simulink model "WP1openloop"  (R2023a)
settings: Solver=ode45  StartTime=0.0  StopTime=100  MaxStep=2  RelTol=1e-14  AbsTol=1e-20
values from neighbouring files (symbols this model uses):
  x1 = x(1)    [WP1.m]    (also in plotSimulationResults.m = x(:, 1))
  x2 = x(2)    [WP1.m]    (also in plotSimulationResults.m = x(:, 2))
settings Model: Creator=giova  LastModifiedBy=giova

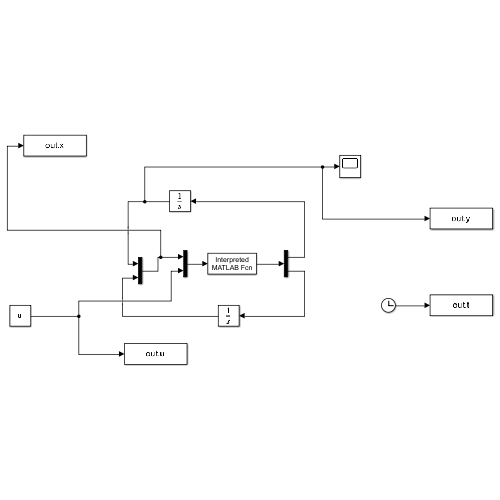
[thumbnail: Simulink's stored preview of the top-level diagram]
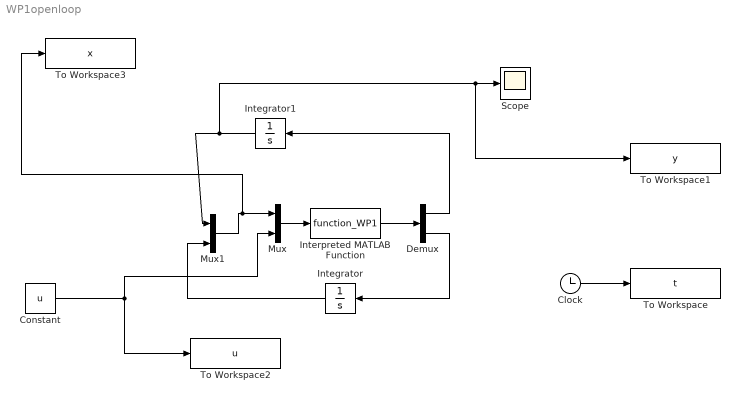
== system WP1openloop ==
  Clock : Clock
  Constant : Constant  Value=u
  Demux : Demux  Outputs=2
  Integrator : Integrator  InitialCondition=x2
  Integrator1 : Integrator  InitialCondition=x1
  Interpreted MATLAB Function : MATLABFcn  MATLABFcn=function_WP1  OutputDimensions=2
  Mux : Mux  Inputs=2
  Mux1 : Mux  Inputs=2
  Scope : Scope
  To Workspace : ToWorkspace  VariableName=t  SampleTime=-1
  To Workspace1 : ToWorkspace  VariableName=y  SampleTime=-1
  To Workspace2 : ToWorkspace  VariableName=u  SampleTime=-1
  To Workspace3 : ToWorkspace  VariableName=x  SampleTime=-1
  wires:
  Demux/2 -> Integrator/1
  Mux/1 -> Interpreted MATLAB Function/1
  Integrator/1 -> Mux1/2
  Demux/1 -> Integrator1/1
  Integrator1/1 -> To Workspace1/1, Scope/1, Mux1/1
  Clock/1 -> To Workspace/1
  Constant/1 -> Mux/2, To Workspace2/1
  Mux1/1 -> To Workspace3/1, Mux/1
  Interpreted MATLAB Function/1 -> Demux/1
